simulink model "diabetes_2slxRaspberry_v3_R2023a"  (R2023a)
settings: Solver=FixedStepAuto  StartTime=0.0  StopTime=100  RelTol=1e-3  EnableMultiTasking=on
StopFcn:
  | plot_results
libraries: raspberrypiNetworklib x2
settings Model: Creator=tsladeche  LastModifiedBy=ryanmccord
settings SolverCC: AlgebraicLoopSolver=TrustRegion  PositivePriorityOrder=on
settings DataIOCC: LimitDataPoints=on  SaveFormat=Array  SignalLoggingSaveFormat=ModelDataLogs  ReturnWorkspaceOutputs=off
settings OptimizationCC: EnhancedBackFolding=on  PassReuseOutputArgsAs=Individual arguments  ExpressionDepthLimit=2147483647  ZeroExternalMemoryAtStartup=off  ZeroInternalMemoryAtStartup=off  MaxStackSize=64  OptimizeBlockOrder=speed  DifferentSizesBufferReuse=on  OptimizationCustomize=off  EfficientTunableParamExpr=on
settings DebuggingCC: UnderspecifiedInitializationDetection=Classic  MergeDetectMultiDrivingBlocksExec=none  SolverPrmCheckMsg=warning  ParameterTunabilityLossMsg=error  FcnCallInpInsideContextMsg=warning  UnconnectedInputMsg=warning  UnconnectedOutputMsg=warning  UnconnectedLineMsg=warning  StateNameClashWarn=warning  SFUnexpectedBacktrackingDiag=warning  SFNoUnconditionalDefaultTransitionDiag=warning  SFExecutionAtInitializationDiag=none  ArithmeticOperatorsInVariantConditions=warning
settings HardwareCC: ProdBitPerPointer=32  ProdBitPerSizeT=32  ProdBitPerPtrDiffT=32  ProdLargestAtomicInteger=Long  ProdLargestAtomicFloat=Double  ProdWordSize=32  ProdLongLongMode=on  ProdHWDeviceType=ARM Compatible->ARM Cortex
settings ModelReferenceCC: PropagateSignalLabelsOutOfModel=off
settings SFSimCC: SimUseLocalCustomCode=off  CustomCodeUndefinedFunction=UseInterfaceOnly
settings RTWCC: Description=Embedded Coder  SystemTargetFile=ert.tlc  HardwareBoard=Raspberry Pi  TLCOptions="-aInlineSetEventsForThisBaseRateFcn=TLC_FALSE -aSuppressMultiTaskScheduler=TLC_FALSE  -aRateBasedStepFcn=0"  TemplateMakefile=ert_default_tmf  RTWUseLocalCustomCode=off  Toolchain=GNU GCC Embedded Linux  BuildConfiguration=Faster Runs
settings CodeAppCC: ForceParamTrailComments=on  IgnoreCustomStorageClasses=off  OperatorAnnotations=on  SimulinkDataObjDesc=on  SFDataObjDesc=on  InsertBlockDesc=on
settings ERTTargetCC: SupportVariableSizeSignals=on  ExtModeTransport=2  ExtModeStaticAlloc=on  ExtModeMexFile=ext_xcp  ExtModeIntrfLevel=Level2 - Open
settings ConfigComp: CovMetricSettings=dw  CovSaveCumulativeToWorkspaceVar=on  CovSaveSingleToWorkspaceVar=on  CovExternalEMLEnable=off

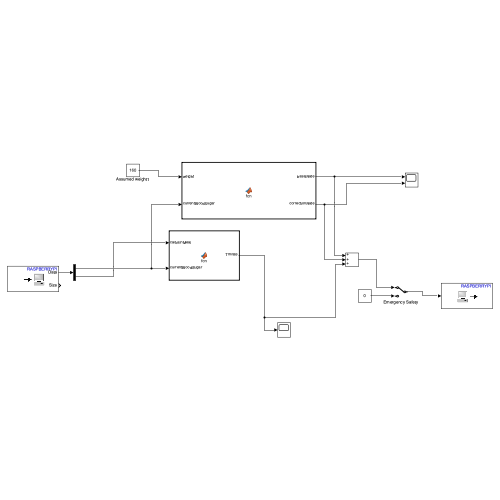
[thumbnail: Simulink's stored preview of the top-level diagram]
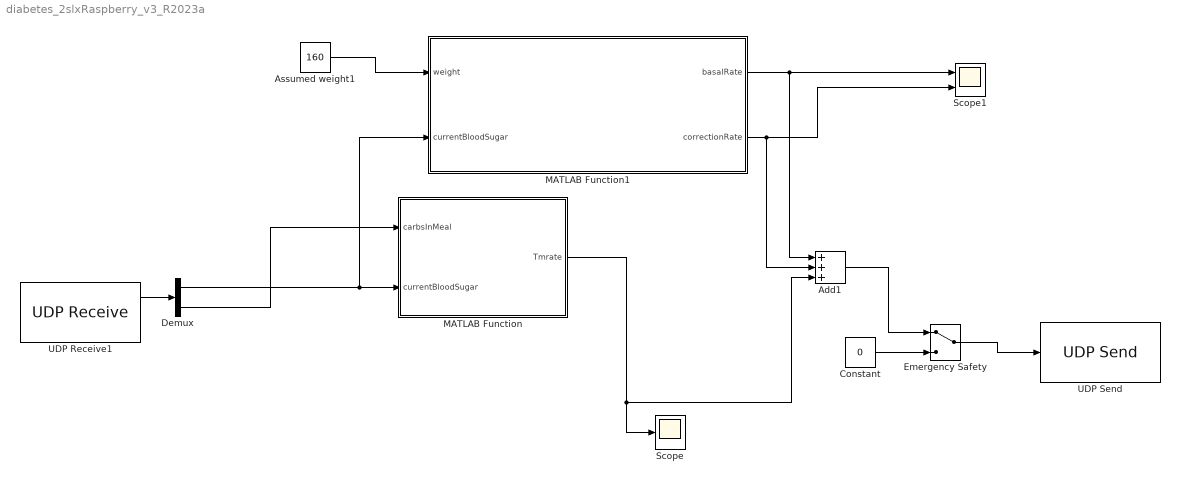
== system diabetes_2slxRaspberry_v3_R2023a ==
  Add1 : Sum  Inputs=+++
  Assumed weight1 : Constant  Value=160
  Constant : Constant  Value=0
  Demux : Demux  Outputs=2
  Emergency Safety : ManualSwitch
  MATLAB Function : MATLAB Function  TreatAsAtomicUnit=on
  MATLAB Function1 : MATLAB Function  TreatAsAtomicUnit=on
  Scope : Scope
  Scope1 : Scope  NumInputPorts=2
  UDP Receive1 : raspberrypiNetworklib/UDP Receive  localURL='0.0.0.0'  localPort=25000  remoteURL='0.0.0.0'  remotePort=-1  recvBufferSize=8192  signalDatatype=uint16  dims=255  isVarSize=off  showBlockingTime=off  blockingTime=0  sampletime=0.01  blockPlatform=Raspberry Pi
  UDP Send : raspberrypiNetworklib/UDP Send  remoteURL='192.168.3.2'  remotePort=26000  localURL='0.0.0.0'  localPortSource=Automatically determine  localPort=-1  sampletime=-1  blockPlatform=Raspberry Pi  separateLengthPort=0
  wires:
  MATLAB Function1/1(basalRate) -> Add1/1, Scope1/1
  MATLAB Function1/2(correctionRate) -> Add1/2, Scope1/2
  Assumed weight1/1 -> MATLAB Function1/1(weight)
  Emergency Safety/1 -> UDP Send/1
  MATLAB Function/1(Tmrate) -> Scope/1, Add1/3
  Add1/1 -> Emergency Safety/1
  Constant/1 -> Emergency Safety/2
  Demux/1 -> MATLAB Function1/2(currentBloodSugar), MATLAB Function/2(currentBloodSugar)
  Demux/2 -> MATLAB Function/1(carbsInMeal)
  UDP Receive1/1 -> Demux/1

== matlab function diabetes_2slxRaspberry_v3_R2023a/MATLAB Function1 ==
  data: weight input; basalRate output; currentBloodSugar input; correctionRate output
function [basalRate, correctionRate]= fcn(weight, currentBloodSugar)

    % Constants
    TARGET_BLOOD_SUGAR = 100; % Target blood sugar level in mg/dl
    CORRECTION_FACTOR_CONSTANT = 1800; % Constant for correction factor calculation

    % Total Daily Insulin Dose (TDI)
    totalDailyInsulin = (weight / 4);

    % Basal/background Insulin Dose
    basalDose = 0.5 * totalDailyInsulin; % 50% of TDI

    % Basal Insulin Delivery Rate per min
    basalRate = basalDose / 24 / 60; % Delivery rate per minute

    % Correction Factor
    correctionFactor = CORRECTION_FACTOR_CONSTANT / totalDailyInsulin;

    % Correction Dose Calculation
    if currentBloodSugar > 120 % High blood sugar state
        correctionDose = (currentBloodSugar - TARGET_BLOOD_SUGAR) / correctionFactor;
    elseif currentBloodSugar < 80 % Low blood sugar state
        basalRate = 0; % Suspend basal insulin delivery
        correctionDose = 0;
    else
        correctionDose = 0; % Normal blood sugar state
    end
    
    correctionRate = correctionDose % Correction Rate per minute
    
end

== matlab function diabetes_2slxRaspberry_v3_R2023a/MATLAB Function ==
  data: carbsInMeal input; currentBloodSugar input; Tmrate output
function Tmrate = fcn(carbsInMeal, currentBloodSugar)

  
 % Constants
    HIGH_BLOOD_SUGAR_CORRECTION_FACTOR = 1/50; % Constant for correction factor calculation
    PRE_MEAL_SUGAR_TAGET = 120;
    INSULIN_TO_CARB_RATIO = 1/10;
    
    %Stage 1: Carbhydrate meal coverage
    CMC = INSULIN_TO_CARB_RATIO * carbsInMeal;
    
    %Stage 2: High Sugar correction Dose;
    deltaSugar = currentBloodSugar - PRE_MEAL_SUGAR_TAGET;
    
    if deltaSugar <= 0
        CD = 0;
    else
        CD = deltaSugar * (HIGH_BLOOD_SUGAR_CORRECTION_FACTOR); 
    end
    
    %Final: Total Meal Insulin Dose
    TM = CD + CMC;
    
    %5 seconds
    if carbsInMeal > 0
        Tmrate = TM / 5 / 60;
    else
        Tmrate = 0;
    end

   

end
